simulink model "Simula"  (R2018a)
settings: Solver=VariableStepAuto  StartTime=0.0  StopTime=12  RelTol=1e-3
values from neighbouring files (symbols this model uses):
  Kf = K(1,:) * F    [Diophantine.m]
  Kgp = K(1,:) * Gp    [Diophantine.m]
undefined symbols (not defined in the file or in its folder): Kr
libraries: cstblocks x1
settings Model: Creator=marcus  LastModifiedBy=marcus

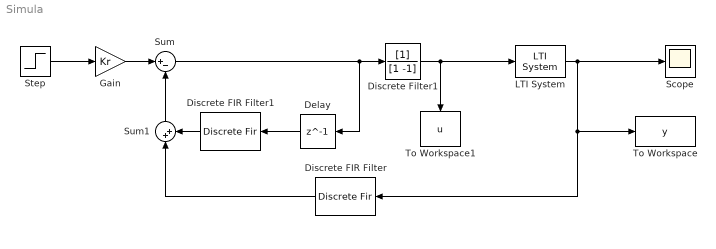
== system Simula ==
  Delay : Delay  DelayLength=1
  Discrete FIR Filter : DiscreteFir  Coefficients=Kf
  Discrete FIR Filter1 : DiscreteFir  Coefficients=Kgp  SampleTime=1
  Discrete Filter1 : DiscreteFilter  Denominator=[1 -1]  SampleTime=1
  Gain : Gain  Gain=Kr
  LTI System : cstblocks/LTI System  sys=P  IC=[]
  Scope : Scope
  Step : Step  Time=0  SampleTime=1
  Sum : Sum  Inputs=|+-
  Sum1 : Sum  Inputs=|++
  To Workspace : ToWorkspace  VariableName=y  SaveFormat=Timeseries  SampleTime=-1
  To Workspace1 : ToWorkspace  VariableName=u  SaveFormat=Timeseries  SampleTime=-1
  wires:
  LTI System/1 -> Scope/1, Discrete FIR Filter/1, To Workspace/1
  Discrete FIR Filter1/1 -> Sum1/2
  Discrete FIR Filter/1 -> Sum1/1
  Sum1/1 -> Sum/2
  Sum/1 -> Discrete Filter1/1, Delay/1
  Step/1 -> Gain/1
  Gain/1 -> Sum/1
  Delay/1 -> Discrete FIR Filter1/1
  Discrete Filter1/1 -> LTI System/1, To Workspace1/1
